simulink model "BNO055_IMU_RegisterMap_AvailableOutputs"  (R2015b)
settings: Solver=VariableStepAuto  StartTime=0.0  StopTime=10.0  RelTol=1e-3
libraries: arduinolib x16
settings Model: Creator=james_000  LastModifiedBy=james_000

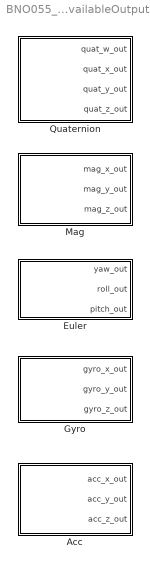
== system BNO055_IMU_RegisterMap_AvailableOutputs ==
  Acc : Subsystem
  Euler : Subsystem
  Gyro : Subsystem
  Mag : Subsystem
  Quaternion : Subsystem

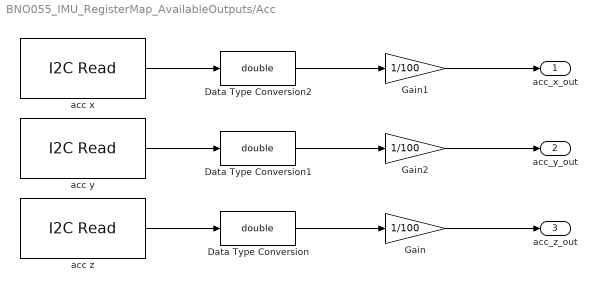
== system BNO055_IMU_RegisterMap_AvailableOutputs/Acc ==
  Data Type Conversion : DataTypeConversion  OutDataTypeStr=double
  Data Type Conversion1 : DataTypeConversion  OutDataTypeStr=double
  Data Type Conversion2 : DataTypeConversion  OutDataTypeStr=double
  Gain : Gain  Gain=1/100
  Gain1 : Gain  Gain=1/100
  Gain2 : Gain  Gain=1/100
  acc x : arduinolib/I2C Read  SlaveAddress_=hex2dec( '28' )  RegisterAddressEnable=on  RegisterAddress_=hex2dec( '08' )  Datatype=uint16  ByteOrder=Big Endian  Datalength_=1  SampleTime_=0.05  blockPlatform=arduino
  acc y : arduinolib/I2C Read  SlaveAddress_=hex2dec( '28' )  RegisterAddressEnable=on  RegisterAddress_=hex2dec( '0A' )  Datatype=uint16  ByteOrder=Big Endian  Datalength_=1  SampleTime_=0.05  blockPlatform=arduino
  acc z : arduinolib/I2C Read  SlaveAddress_=hex2dec( '28' )  RegisterAddressEnable=on  RegisterAddress_=hex2dec( '0C' )  Datatype=uint16  ByteOrder=Big Endian  Datalength_=1  SampleTime_=0.05  blockPlatform=arduino
  acc_x_out : Outport
  acc_y_out : Outport  Port=2
  acc_z_out : Outport  Port=3
  wires:
  acc y/1 -> Data Type Conversion1/1
  acc z/1 -> Data Type Conversion/1
  acc x/1 -> Data Type Conversion2/1
  Data Type Conversion2/1 -> Gain1/1
  Data Type Conversion1/1 -> Gain2/1
  Data Type Conversion/1 -> Gain/1
  Gain1/1 -> acc_x_out/1
  Gain2/1 -> acc_y_out/1
  Gain/1 -> acc_z_out/1

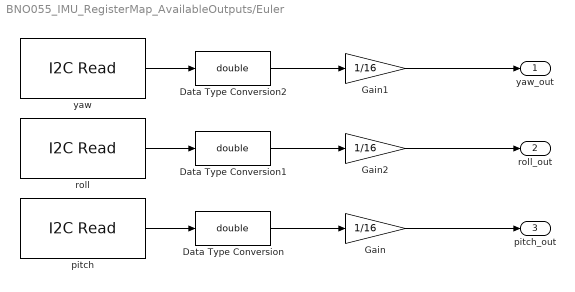
== system BNO055_IMU_RegisterMap_AvailableOutputs/Euler ==
  Data Type Conversion : DataTypeConversion  OutDataTypeStr=double
  Data Type Conversion1 : DataTypeConversion  OutDataTypeStr=double
  Data Type Conversion2 : DataTypeConversion  OutDataTypeStr=double
  Gain : Gain  Gain=1/16
  Gain1 : Gain  Gain=1/16
  Gain2 : Gain  Gain=1/16
  pitch : arduinolib/I2C Read  SlaveAddress_=hex2dec( '28' )  RegisterAddressEnable=on  RegisterAddress_=hex2dec( '1E' )  Datatype=uint16  ByteOrder=Big Endian  Datalength_=1  SampleTime_=0.05  blockPlatform=arduino
  roll : arduinolib/I2C Read  SlaveAddress_=hex2dec( '28' )  RegisterAddressEnable=on  RegisterAddress_=hex2dec( '1C' )  Datatype=uint16  ByteOrder=Big Endian  Datalength_=1  SampleTime_=0.05  blockPlatform=arduino
  yaw : arduinolib/I2C Read  SlaveAddress_=hex2dec( '28' )  RegisterAddressEnable=on  RegisterAddress_=hex2dec( '1A' )  Datatype=uint16  ByteOrder=Big Endian  Datalength_=1  SampleTime_=0.05  blockPlatform=arduino
  yaw_out : Outport
  roll_out : Outport  Port=2
  pitch_out : Outport  Port=3
  wires:
  pitch/1 -> Data Type Conversion/1
  yaw/1 -> Data Type Conversion2/1
  roll/1 -> Data Type Conversion1/1
  Data Type Conversion/1 -> Gain/1
  Data Type Conversion1/1 -> Gain2/1
  Data Type Conversion2/1 -> Gain1/1
  Gain/1 -> pitch_out/1
  Gain2/1 -> roll_out/1
  Gain1/1 -> yaw_out/1

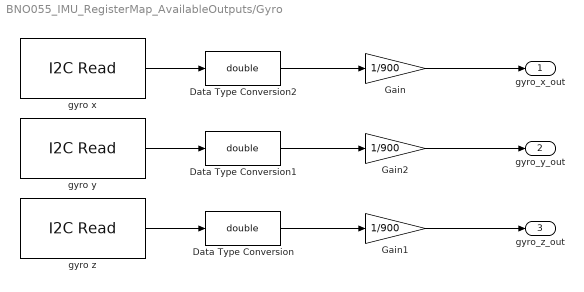
== system BNO055_IMU_RegisterMap_AvailableOutputs/Gyro ==
  Data Type Conversion : DataTypeConversion  OutDataTypeStr=double
  Data Type Conversion1 : DataTypeConversion  OutDataTypeStr=double
  Data Type Conversion2 : DataTypeConversion  OutDataTypeStr=double
  Gain : Gain  Gain=1/900
  Gain1 : Gain  Gain=1/900
  Gain2 : Gain  Gain=1/900
  gyro x : arduinolib/I2C Read  SlaveAddress_=hex2dec( '28' )  RegisterAddressEnable=on  RegisterAddress_=hex2dec( '26' )  Datatype=uint16  ByteOrder=Big Endian  Datalength_=1  SampleTime_=0.05  blockPlatform=arduino
  gyro y : arduinolib/I2C Read  SlaveAddress_=hex2dec( '28' )  RegisterAddressEnable=on  RegisterAddress_=hex2dec( '26' )  Datatype=uint16  ByteOrder=Big Endian  Datalength_=1  SampleTime_=0.05  blockPlatform=arduino
  gyro z : arduinolib/I2C Read  SlaveAddress_=hex2dec( '28' )  RegisterAddressEnable=on  RegisterAddress_=hex2dec( '26' )  Datatype=uint16  ByteOrder=Big Endian  Datalength_=1  SampleTime_=0.05  blockPlatform=arduino
  gyro_x_out : Outport
  gyro_y_out : Outport  Port=2
  gyro_z_out : Outport  Port=3
  wires:
  gyro x/1 -> Data Type Conversion2/1
  gyro z/1 -> Data Type Conversion/1
  gyro y/1 -> Data Type Conversion1/1
  Data Type Conversion1/1 -> Gain2/1
  Data Type Conversion2/1 -> Gain/1
  Data Type Conversion/1 -> Gain1/1
  Gain1/1 -> gyro_z_out/1
  Gain2/1 -> gyro_y_out/1
  Gain/1 -> gyro_x_out/1

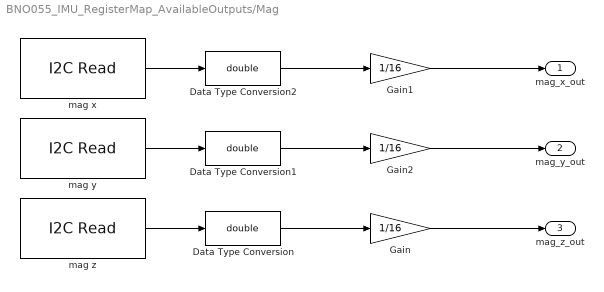
== system BNO055_IMU_RegisterMap_AvailableOutputs/Mag ==
  Data Type Conversion : DataTypeConversion  OutDataTypeStr=double
  Data Type Conversion1 : DataTypeConversion  OutDataTypeStr=double
  Data Type Conversion2 : DataTypeConversion  OutDataTypeStr=double
  Gain : Gain  Gain=1/16
  Gain1 : Gain  Gain=1/16
  Gain2 : Gain  Gain=1/16
  mag x : arduinolib/I2C Read  SlaveAddress_=hex2dec( '28' )  RegisterAddressEnable=on  RegisterAddress_=hex2dec( '0E' )  Datatype=uint16  ByteOrder=Big Endian  Datalength_=1  SampleTime_=0.05  blockPlatform=arduino
  mag y : arduinolib/I2C Read  SlaveAddress_=hex2dec( '28' )  RegisterAddressEnable=on  RegisterAddress_=hex2dec( '10' )  Datatype=uint16  ByteOrder=Big Endian  Datalength_=1  SampleTime_=0.05  blockPlatform=arduino
  mag z : arduinolib/I2C Read  SlaveAddress_=hex2dec( '28' )  RegisterAddressEnable=on  RegisterAddress_=hex2dec( '12' )  Datatype=uint16  ByteOrder=Big Endian  Datalength_=1  SampleTime_=0.05  blockPlatform=arduino
  mag_x_out : Outport
  mag_y_out : Outport  Port=2
  mag_z_out : Outport  Port=3
  wires:
  mag z/1 -> Data Type Conversion/1
  mag x/1 -> Data Type Conversion2/1
  mag y/1 -> Data Type Conversion1/1
  Data Type Conversion2/1 -> Gain1/1
  Data Type Conversion1/1 -> Gain2/1
  Data Type Conversion/1 -> Gain/1
  Gain1/1 -> mag_x_out/1
  Gain2/1 -> mag_y_out/1
  Gain/1 -> mag_z_out/1

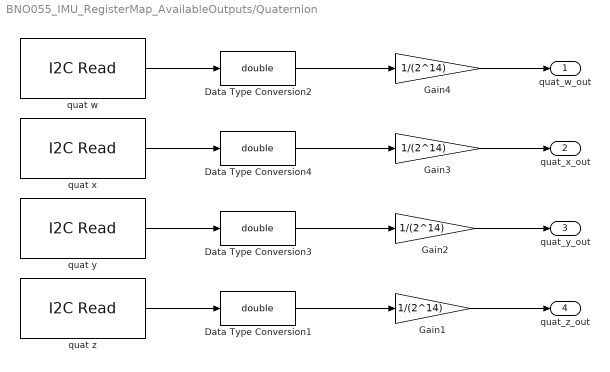
== system BNO055_IMU_RegisterMap_AvailableOutputs/Quaternion ==
  Data Type Conversion{1..4} (4 alike) : DataTypeConversion  OutDataTypeStr=double
  Gain{1..4} (4 alike) : Gain  Gain=1/(2^14)
  quat w : arduinolib/I2C Read  SlaveAddress_=hex2dec( '28' )  RegisterAddressEnable=on  RegisterAddress_=hex2dec( '20' )  Datatype=uint16  ByteOrder=Big Endian  Datalength_=1  SampleTime_=0.05  blockPlatform=arduino
  quat x : arduinolib/I2C Read  SlaveAddress_=hex2dec( '28' )  RegisterAddressEnable=on  RegisterAddress_=hex2dec( '22' )  Datatype=uint16  ByteOrder=Big Endian  Datalength_=1  SampleTime_=0.05  blockPlatform=arduino
  quat y : arduinolib/I2C Read  SlaveAddress_=hex2dec( '28' )  RegisterAddressEnable=on  RegisterAddress_=hex2dec( '24' )  Datatype=uint16  ByteOrder=Big Endian  Datalength_=1  SampleTime_=0.05  blockPlatform=arduino
  quat z : arduinolib/I2C Read  SlaveAddress_=hex2dec( '28' )  RegisterAddressEnable=on  RegisterAddress_=hex2dec( '26' )  Datatype=uint16  ByteOrder=Big Endian  Datalength_=1  SampleTime_=0.05  blockPlatform=arduino
  quat_w_out : Outport
  quat_x_out : Outport  Port=2
  quat_y_out : Outport  Port=3
  quat_z_out : Outport  Port=4
  wires:
  quat x/1 -> Data Type Conversion4/1
  quat w/1 -> Data Type Conversion2/1
  quat y/1 -> Data Type Conversion3/1
  quat z/1 -> Data Type Conversion1/1
  Data Type Conversion2/1 -> Gain4/1
  Data Type Conversion4/1 -> Gain3/1
  Data Type Conversion3/1 -> Gain2/1
  Data Type Conversion1/1 -> Gain1/1
  Gain4/1 -> quat_w_out/1
  Gain3/1 -> quat_x_out/1
  Gain2/1 -> quat_y_out/1
  Gain1/1 -> quat_z_out/1
